simulink model "BVH2_App_Layer"  (Simulink 5.1)
settings: Solver=ode45  StartTime=0.0  StopTime=10.0  RelTol=1e-3
PreLoadFcn:
  | if exist('tl_preloadfcn','file'), tl_preloadfcn(gcs,95); end
PostLoadFcn:
  | if exist('tl_postloadfcn','file'), tl_postloadfcn(gcs,95); end
InitFcn:
  | if exist('tlds_start','file'), tlds_start(gcs); end
undefined symbols (not defined in the file): built, constant, Constant, DiscreteIntegrator, Gain, in, Logic, Product, Saturate, Sum, Switch
libraries: tllib x71, simulink x1
(part 1 of 4)
PreSaveFcn:
  | if exist('tl_presavefcn','file'), tl_presavefcn(gcs); end
CloseFcn:
  | rtwprivate ssgencode ModelCloseRequest BVH2_App_Layer
settings Model: LastModifiedBy=adequatrebarbes  BooleanDataType=on  ProdHWDeviceType=Microprocessor  RTWOptions="-aEnforceIntegerDowncast=1 -aExtMode=0 -aExtModeTesting=0 -aFoldNonRolledExpr=1 -aForceParamTrailComments=0 -aGenerateComments=1 -aGenerateReport=0 -aIgnoreCustomStorageClasses=0 -aIncDataTypeInIds=0 -aIncHierarchyInIds=0 -aInlineInvariantSignals=0 -aInlinedPrmAccess=\"Literals\" -aLocalBlockOutputs=1 -aLogVarNameModifier=\"rt_\" -aMaxRTWIdLen=31 -aPrefixModelToSubsysFcnNames=1 -aRTWVerbose=1 -aRollThreshold=5 -aShowEliminatedStatements=0"  TL_MAIN_DATA=struct('date',736137.66153059,'maxnumsimulations',10,'codeopt',struct('inliningthreshold',6,'target',['Generic ANSI-C'],'assembler',0,'optlevel',2,'linebreaklimit',100,'stateactcodinglimit',5,'functionsfor64bitops',1,'sections',1,'sfbitfields',1,'globalbitfields',0,'sharefunctions',0,'noinitstozero',0,'limidentlength',1,'decimals',1,'separatesearch',0,'cleancode',1,'optimizedbooltype',1,'keepsaturation',0,'extvarsharing',0,'outputstylefile','cconfig.xml','rootstylesheet','TL_CSourceCodeSS.xsl'),'frameopt',struct('exectime',1,'stacksize',1,'simconfig',['default EVM'],'targettimeout',1,'mexargs','-g','tcargs',''),'logopt',struct('plotinterval',0.1,'globalloggingmode',1),'export',struct('directory','.\export','sysfiles',1,'docfiles',0,'tools',0),'codecoveragelevel',0,'asapscript','asap2_all_in_one','docscript','tldoc_default','rtos',struct('enablemultirate',0,'currentrtos',['generic RTOS'],'autopriority',0,'autoinitalarm',1,'alarminitwithrestart',1,'alarmactivationkind',1,'alarmstartoffset',0))

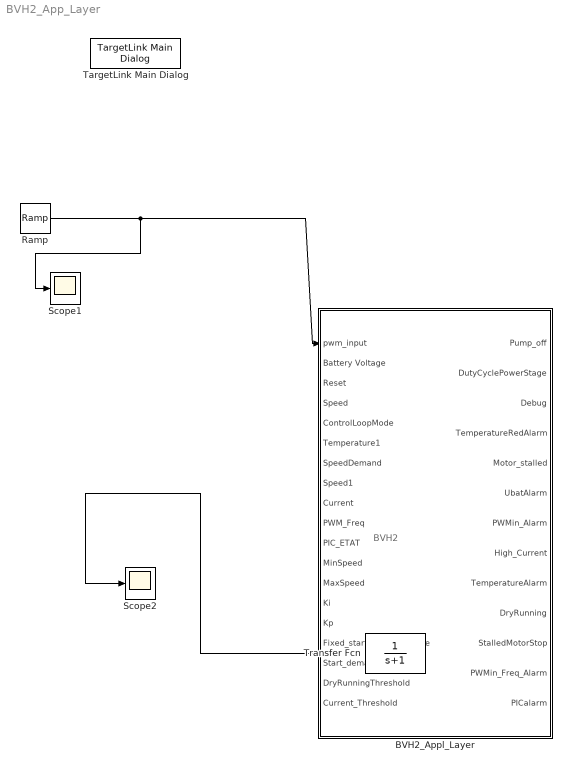
== system BVH2_App_Layer ==
  note: BVH2
  BVH2_Appl_Layer : Subsystem  Tag=TargetLink Simulation Frame
      settings: CopyFcn=if exist('tl_copyfcn','file'), tl_copyfcn(gcbh); end  NameChangeFcn=if exist('tl_framenamechangefcn','file'), tl_framenamechangefcn(gcbh); end  OpenFcn=if exist('open_tlsubsystem','file'), open_tlsubsystem(gcbh); end
      mask Type: TL_SimFrame
      mask Display: disp('TargetLink\nModel-\nin-the-loop\nmode')
  Ramp : simulink/Sources/Ramp  slope=10  start=0  X0=0
  Scope1 : Scope
  Scope2 : Scope
      settings: SaveName=ScopeData2
  TargetLink Main Dialog : tllib/TargetLink Main Dialog  flp_block=none
  Transfer Fcn : TransferFcn  Orientation=left  Denominator=[1 1]
  wires:
  Ramp/1 -> BVH2_Appl_Layer/1(pwm_input), Scope1/1
  Transfer Fcn/1 -> Scope2/1

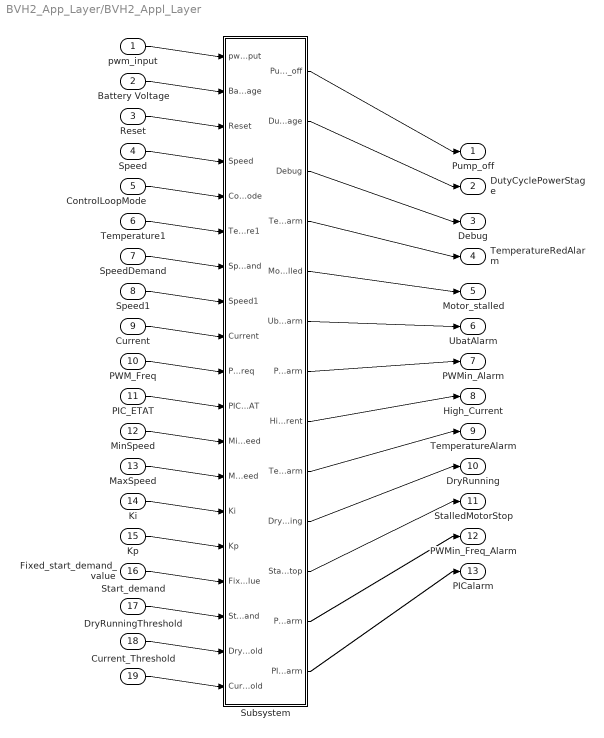
== system BVH2_App_Layer/BVH2_Appl_Layer ==
  pwm_input : Inport  PortDimensions=1  SampleTime=0.01
  Battery Voltage : Inport  Port=2  PortDimensions=1  SampleTime=0.01
  Reset : Inport  Port=3  SampleTime=0.01
  Speed : Inport  Port=4  PortDimensions=1  SampleTime=0.01
  ControlLoopMode : Inport  Port=5  PortDimensions=1  SampleTime=0.01
  Temperature1 : Inport  Port=6  PortDimensions=1  SampleTime=0.01
  SpeedDemand : Inport  Port=7  PortDimensions=1  SampleTime=0.01
  Speed1 : Inport  Port=8  PortDimensions=1  SampleTime=0.01
  Current : Inport  Port=9  PortDimensions=1  SampleTime=0.01
  PWM_Freq : Inport  Port=10  PortDimensions=1  SampleTime=0.01
  PIC_ETAT : Inport  Port=11  PortDimensions=1  SampleTime=0.01
  MinSpeed : Inport  Port=12  SampleTime=0.01
  MaxSpeed : Inport  Port=13  SampleTime=0.01
  Ki : Inport  Port=14  SampleTime=0.01
  Kp : Inport  Port=15  SampleTime=0.01
  Fixed_start_demand_value : Inport  Port=16  PortDimensions=1  SampleTime=0.01
  Start_demand : Inport  Port=17  PortDimensions=1  SampleTime=0.01
  DryRunningThreshold : Inport  Port=18  PortDimensions=1  SampleTime=0.01
  Current_Threshold : Inport  Port=19  PortDimensions=1  SampleTime=0.01
  Subsystem : Subsystem  Tag=struct('sfcnName','Control_sf','subFunction','','srcSubsystem','')
      settings: OpenFcn=warndlg(get_param(gcb,'MaskHelp'),'Serious Warning');
      mask Type: TL_Enable
      mask Help: This subsystem keeps the TargetLink subsystem (subsystem with TargetLink blocks for production code generation), and is needed for the TargetLink simulation frame to work properly. DO NOT DELETE OR MODIFY IT!
  Pump_off : Outport
  DutyCyclePowerStage : Outport  Port=2
  Debug : Outport  Port=3
  TemperatureRedAlarm : Outport  Port=4
  Motor_stalled : Outport  Port=5
  UbatAlarm : Outport  Port=6
  PWMin_Alarm : Outport  Port=7
  High_Current : Outport  Port=8
  TemperatureAlarm : Outport  Port=9
  DryRunning : Outport  Port=10
  StalledMotorStop : Outport  Port=11
  PWMin_Freq_Alarm : Outport  Port=12
  PICalarm : Outport  Port=13
  wires:
  pwm_input/1 -> Subsystem/1(pwm_input)
  Battery Voltage/1 -> Subsystem/2(Battery Voltage)
  Reset/1 -> Subsystem/3(Reset)
  Speed/1 -> Subsystem/4(Speed)
  ControlLoopMode/1 -> Subsystem/5(ControlLoopMode)
  Temperature1/1 -> Subsystem/6(Temperature1)
  SpeedDemand/1 -> Subsystem/7(SpeedDemand)
  Speed1/1 -> Subsystem/8(Speed1)
  Current/1 -> Subsystem/9(Current)
  PWM_Freq/1 -> Subsystem/10(PWM_Freq)
  PIC_ETAT/1 -> Subsystem/11(PIC_ETAT)
  MinSpeed/1 -> Subsystem/12(MinSpeed)
  MaxSpeed/1 -> Subsystem/13(MaxSpeed)
  Ki/1 -> Subsystem/14(Ki)
  Kp/1 -> Subsystem/15(Kp)
  Fixed_start_demand_value/1 -> Subsystem/16(Fixed_start_demand_value)
  Start_demand/1 -> Subsystem/17(Start_demand)
  DryRunningThreshold/1 -> Subsystem/18(DryRunningThreshold)
  Current_Threshold/1 -> Subsystem/19(Current_Threshold)
  Subsystem/1(Pump_off) -> Pump_off/1
  Subsystem/2(DutyCyclePowerStage) -> DutyCyclePowerStage/1
  Subsystem/3(Debug) -> Debug/1
  Subsystem/4(TemperatureRedAlarm) -> TemperatureRedAlarm/1
  Subsystem/5(Motor_stalled) -> Motor_stalled/1
  Subsystem/6(UbatAlarm) -> UbatAlarm/1
  Subsystem/7(PWMin_Alarm) -> PWMin_Alarm/1
  Subsystem/8(High_Current) -> High_Current/1
  Subsystem/9(TemperatureAlarm) -> TemperatureAlarm/1
  Subsystem/10(DryRunning) -> DryRunning/1
  Subsystem/11(StalledMotorStop) -> StalledMotorStop/1
  Subsystem/12(PWMin_Freq_Alarm) -> PWMin_Freq_Alarm/1
  Subsystem/13(PICalarm) -> PICalarm/1

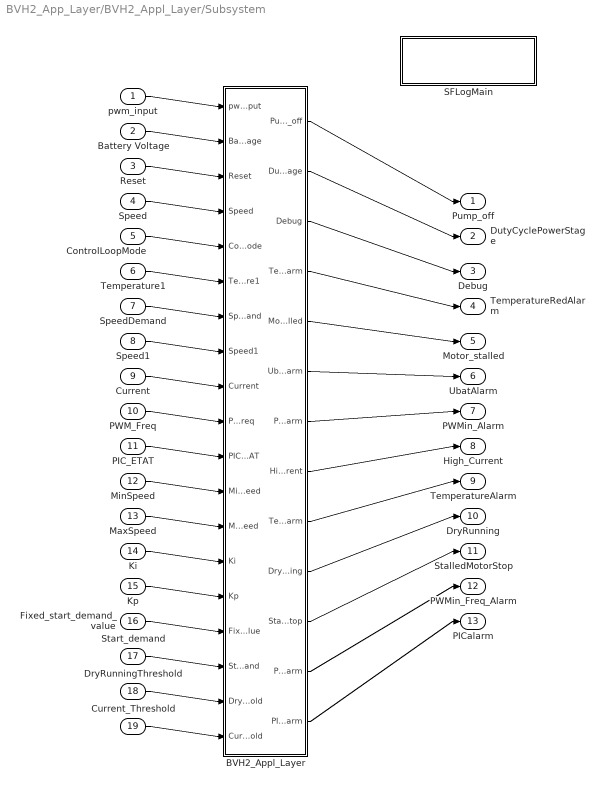
== system BVH2_App_Layer/BVH2_Appl_Layer/Subsystem ==
  pwm_input : Inport  PortDimensions=1  SampleTime=0.01
  Battery Voltage : Inport  Port=2  PortDimensions=1  SampleTime=0.01
  Reset : Inport  Port=3  SampleTime=0.01
  Speed : Inport  Port=4  PortDimensions=1  SampleTime=0.01
  ControlLoopMode : Inport  Port=5  PortDimensions=1  SampleTime=0.01
  Temperature1 : Inport  Port=6  PortDimensions=1  SampleTime=0.01
  SpeedDemand : Inport  Port=7  PortDimensions=1  SampleTime=0.01
  Speed1 : Inport  Port=8  PortDimensions=1  SampleTime=0.01
  Current : Inport  Port=9  PortDimensions=1  SampleTime=0.01
  PWM_Freq : Inport  Port=10  PortDimensions=1  SampleTime=0.01
  PIC_ETAT : Inport  Port=11  PortDimensions=1  SampleTime=0.01
  MinSpeed : Inport  Port=12  SampleTime=0.01
  MaxSpeed : Inport  Port=13  SampleTime=0.01
  Ki : Inport  Port=14  SampleTime=0.01
  Kp : Inport  Port=15  SampleTime=0.01
  Fixed_start_demand_value : Inport  Port=16  PortDimensions=1  SampleTime=0.01
  Start_demand : Inport  Port=17  PortDimensions=1  SampleTime=0.01
  DryRunningThreshold : Inport  Port=18  PortDimensions=1  SampleTime=0.01
  Current_Threshold : Inport  Port=19  PortDimensions=1  SampleTime=0.01
  BVH2_Appl_Layer : Subsystem  Tag=MIL Subsystem  Description=b
      settings: CopyFcn=if exist('tl_copyfcn','file'), tl_copyfcn(gcbh); end  NameChangeFcn=if exist('tl_namechangefcn','file'), tl_namechangefcn(gcbh); end  DestroyFcn=if exist('update_tl_main_dlg','file'), update_tl_main_dlg('TL_subs_display'); end
  SFLogMain : Subsystem
      mask Type: TL_StateflowLoggingMain
      mask Display:
      | plot([0 0 1 1 0 0 1 1 0],[0 1 1 0 0 0.05 0.05 0.95 0.95]);
      | disp('Stateflow Logging Main\nDO NOT DELETE')
  Pump_off : Outport
  DutyCyclePowerStage : Outport  Port=2
  Debug : Outport  Port=3
  TemperatureRedAlarm : Outport  Port=4
  Motor_stalled : Outport  Port=5
  UbatAlarm : Outport  Port=6
  PWMin_Alarm : Outport  Port=7
  High_Current : Outport  Port=8
  TemperatureAlarm : Outport  Port=9
  DryRunning : Outport  Port=10
  StalledMotorStop : Outport  Port=11
  PWMin_Freq_Alarm : Outport  Port=12
  PICalarm : Outport  Port=13
  wires:
  pwm_input/1 -> BVH2_Appl_Layer/1(pwm_input)
  Battery Voltage/1 -> BVH2_Appl_Layer/2(Battery Voltage)
  Reset/1 -> BVH2_Appl_Layer/3(Reset)
  Speed/1 -> BVH2_Appl_Layer/4(Speed)
  ControlLoopMode/1 -> BVH2_Appl_Layer/5(ControlLoopMode)
  Temperature1/1 -> BVH2_Appl_Layer/6(Temperature1)
  SpeedDemand/1 -> BVH2_Appl_Layer/7(SpeedDemand)
  Speed1/1 -> BVH2_Appl_Layer/8(Speed1)
  Current/1 -> BVH2_Appl_Layer/9(Current)
  PWM_Freq/1 -> BVH2_Appl_Layer/10(PWM_Freq)
  PIC_ETAT/1 -> BVH2_Appl_Layer/11(PIC_ETAT)
  MinSpeed/1 -> BVH2_Appl_Layer/12(MinSpeed)
  MaxSpeed/1 -> BVH2_Appl_Layer/13(MaxSpeed)
  Ki/1 -> BVH2_Appl_Layer/14(Ki)
  Kp/1 -> BVH2_Appl_Layer/15(Kp)
  Fixed_start_demand_value/1 -> BVH2_Appl_Layer/16(Fixed_start_demand_value)
  Start_demand/1 -> BVH2_Appl_Layer/17(Start_demand)
  DryRunningThreshold/1 -> BVH2_Appl_Layer/18(DryRunningThreshold)
  Current_Threshold/1 -> BVH2_Appl_Layer/19(Current_Threshold)
  BVH2_Appl_Layer/1(Pump_off) -> Pump_off/1
  BVH2_Appl_Layer/2(DutyCyclePowerStage) -> DutyCyclePowerStage/1
  BVH2_Appl_Layer/3(Debug) -> Debug/1
  BVH2_Appl_Layer/4(TemperatureRedAlarm) -> TemperatureRedAlarm/1
  BVH2_Appl_Layer/5(Motor_stalled) -> Motor_stalled/1
  BVH2_Appl_Layer/6(UbatAlarm) -> UbatAlarm/1
  BVH2_Appl_Layer/7(PWMin_Alarm) -> PWMin_Alarm/1
  BVH2_Appl_Layer/8(High_Current) -> High_Current/1
  BVH2_Appl_Layer/9(TemperatureAlarm) -> TemperatureAlarm/1
  BVH2_Appl_Layer/10(DryRunning) -> DryRunning/1
  BVH2_Appl_Layer/11(StalledMotorStop) -> StalledMotorStop/1
  BVH2_Appl_Layer/12(PWMin_Freq_Alarm) -> PWMin_Freq_Alarm/1
  BVH2_Appl_Layer/13(PICalarm) -> PICalarm/1
